simulink model "Model_Slides"  (R2021b)
settings: Solver=VariableStepAuto  StartTime=0.0  StopTime=inf  RelTol=1e-3
model workspace (MAT data in the model file):
  firstWarning = 1
  originalScenarioChecksum = '114339432DE22364D47BB28FC96DC10C'
undefined symbols (not defined in the file): Acceleration, ActorID, AngularVelocity, curvature, DefaultGear, DEND_B, DEND_S, DEND_T, direction, driving, gradbp, LF, LR, matlabshared, MAX_BRAKE, MAX_STEER, MAX_TORQUE, MCAR, MIN_BRAKE, MIN_STEER, MIN_TORQUE, NUMD_B, NUMD_S, NUMD_T, Pitch, Position, psi_o, R, Roll, RRdamp, scenario, SceneInfo, sigbuilder_block, STEER_RATIO, stopSign_ID, Tdead, thetaRefs, TL_ID, TrackWidth, Ts, ts, Vdead, Velocity, X_o, xRef2s, Y_o, Yaw, yRef2s
libraries: drivingscenarioandsensors x8, drivingvehiclecontroller x2, simulink x2, trackingutilitieslib x2, mpcadaslib x1, simulink_extras x1, drivinglib x1, autolibshared x1, vehdynlibviscommon x1, vehdynlibsteering x1
(part 1 of 2)
settings Model: Creator=akshran  LastModifiedBy=moham

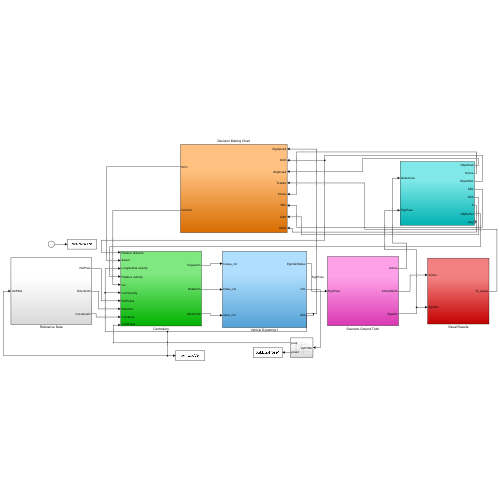
[thumbnail: Simulink's stored preview of the top-level diagram]
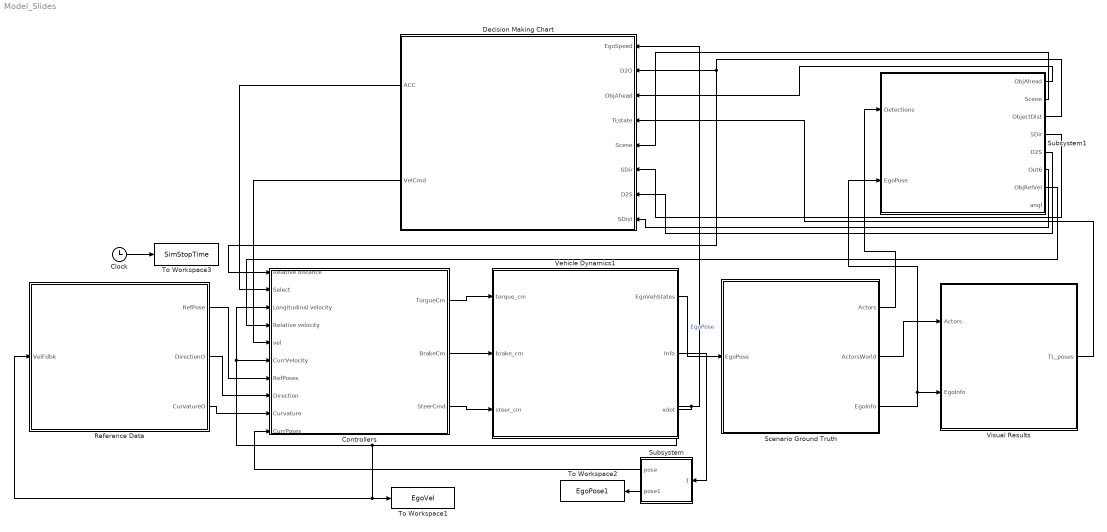
== system Model_Slides ==
  Clock : Clock
  Controllers : Subsystem
  Decision Making Chart : Subsystem
  Reference Data : Subsystem  VariantControl=Stanley
  Scenario Ground Truth : Subsystem
  Subsystem : Subsystem
  Subsystem1 : Subsystem
  To Workspace1 : ToWorkspace  VariableName=EgoVel  SampleTime=-1
      settings: Save2DSignal=2-D array (concatenate along first dimension)
  To Workspace2 : ToWorkspace  VariableName=EgoPose1  SampleTime=-1
      settings: Save2DSignal=2-D array (concatenate along first dimension)
  To Workspace3 : ToWorkspace  VariableName=SimStopTime  SampleTime=-1
      settings: Save2DSignal=2-D array (concatenate along first dimension)
  Vehicle Dynamics1 : Subsystem
  Visual Results : Subsystem
  wires:
  Vehicle Dynamics1/2(Info) -> Subsystem/1(VehFdbk)
  Clock/1 -> To Workspace3/1
  Vehicle Dynamics1/3(xdot) -> Reference Data/1(VelFdbk), To Workspace1/1, Controllers/6(CurrVelocity), Controllers/3(Longitudinal velocity), Decision Making Chart/1(EgoSpeed)
  Subsystem/2(pose1) -> To Workspace2/1
  Reference Data/1(RefPose) -> Controllers/7(RefPoses)
  Reference Data/2(DirectionO) -> Controllers/8(Direction)
  Reference Data/3(CurvatureO) -> Controllers/9(Curvature)
  Subsystem/1(pose) -> Controllers/10(CurrPoses)
  Controllers/1(TorgueCm) -> Vehicle Dynamics1/1(torque_cm)
  Controllers/2(BrakeCm) -> Vehicle Dynamics1/2(brake_cm)
  Controllers/3(SteerCmd) -> Vehicle Dynamics1/3(steer_cm)
  Visual Results/1(TL_poses) -> Decision Making Chart/4(TLstate)
  Decision Making Chart/1(ACC) -> Controllers/2(Select)
  Decision Making Chart/2(VelCmd) -> Controllers/5(vel)
  Subsystem1/3(ObjectDist) -> Controllers/1(Relative distance), Decision Making Chart/2(D2O)
  Subsystem1/1(ObjAhead) -> Decision Making Chart/3(ObjAhead)
  Subsystem1/2(Scene) -> Decision Making Chart/5(Scene)
  Subsystem1/4(SDir) -> Decision Making Chart/6(SDir)
  Subsystem1/5(D2S) -> Decision Making Chart/7(D2S)
  Subsystem1/6(Out6) -> Decision Making Chart/8(SDist)
  Subsystem1/7(ObjRelVel) -> Controllers/4(Relative velocity)
  Vehicle Dynamics1/1(EgoVehStates) -> Scenario Ground Truth/1(EgoPose)  "EgoPose"
  Scenario Ground Truth/1(Actors) -> Subsystem1/1(Detections)
  Scenario Ground Truth/2(ActorsWorld) -> Visual Results/1(Actors)
  Scenario Ground Truth/3(EgoInfo) -> Subsystem1/2(EgoPose), Visual Results/2(EgoInfo)

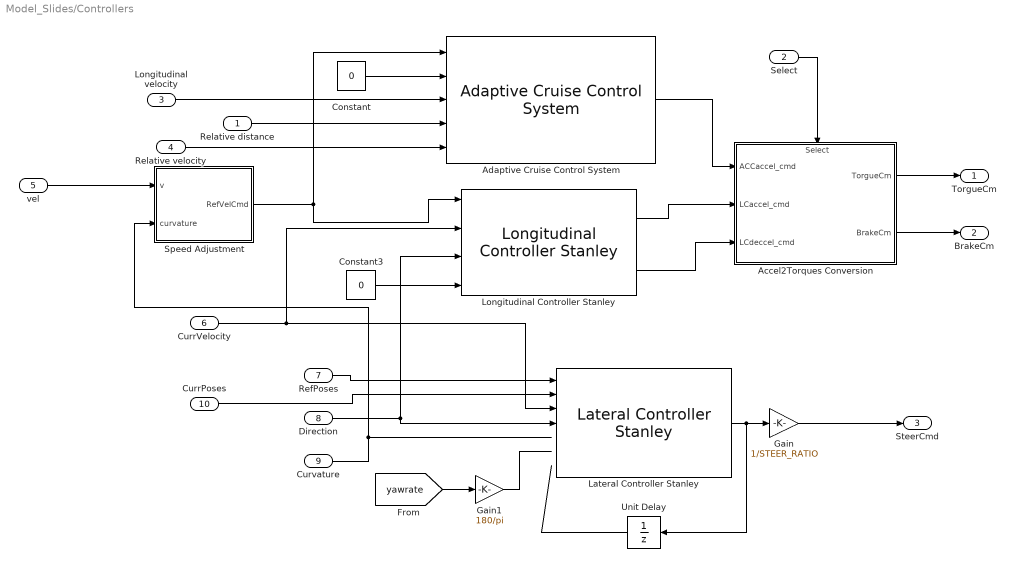
== system Model_Slides/Controllers ==
  Relative distance : Inport
  Select : Inport  Port=2
  Longitudinal velocity : Inport  Port=3
  Relative velocity : Inport  Port=4
  vel : Inport  Port=5
  CurrVelocity : Inport  Port=6
  RefPoses : Inport  Port=7
  Direction : Inport  Port=8
  Curvature : Inport  Port=9
  CurrPoses : Inport  Port=10
  Accel2Torques Conversion : Subsystem
      settings: PortSchema="{\"entries\":[{\"content\":{\"sides\":[{\"content\":{\"connectorIds\":[\"In1\",\"In2\",\"In3\"]},\"type\":\"ConnectorPlacement.EquallySpacedRectSide\",\"uuid\":\"a23b1a10-3bcb-40a0-900c-c9a3f160b173\"},{\"content\":{\"connectorIds\":[\"Out1\",\"Out2\"],\"side\":\"RIGHT\"},\"type\":\"ConnectorPlacement.EquallySpacedRectSide\",\"uuid\":\"88840b66-912f-4184-aeec-297642319416\"},{\"content\":{\"connectorIds\":[\"In4\"],\"side\":\"TOP\"},\"type\":\"ConnectorPlacement.EquallySpacedRectSide\",\"uuid\":\"37a03ca9-b065-473e-b290-3b07703c6005\"}]},\"type\":\"ConnectorPlacement.EquallySpacedConnector\",\"uuid\":\"5bfc7c71-8f7a-4cba-a168-7eeca22a2fcb\"}],\"packageUris\":[\"http://schema.mathworks.com/mf0/Connector/R2020b\"],\"version\":\"1.0\"}"
  Adaptive Cruise Control System : mpcadaslib/Adaptive Cruise Control System  EgoModel=tf(1,[0.5,1,0])  InitialEgoVelocity=0  DefaultSpacing=10  MaxVelocity=50  MinAcceleration=-6  amin_ext=off  MaxAcceleration=6  amax_ext=off  Ts=0.1  PredictionHorizon=30  ControllerBehavior=0.5  suboptimal=off  maxiter=10  datatypeopt=double  optmode=off  trackmode=off
  Constant : Constant  Value=0
  Constant3 : Constant  Value=0
  Gain : Gain  Gain=1/STEER_RATIO
  Gain1 : Gain  Gain=180/pi
  Lateral Controller Stanley : drivingvehiclecontroller/Lateral Controller Stanley  ModelType=Dynamic bicycle model  PositionGainF=2.5  PositionGainR=2.5  YawRateGain=0.2  DelayGain=0.2  VehicleMass=MCAR  Lf=LF  Lr=LR  TireStiffness=5e3  Wheelbase=3  MaxSteeringAngle=80
      settings: SourceProductBaseCode=DR
  Longitudinal Controller Stanley : drivingvehiclecontroller/Longitudinal Controller Stanley  Kp=10  Ki=0.1  SampleTime=0.05  MaxAcceleration=40  MaxDeceleration=40
      settings: SourceProductBaseCode=DR
  Speed Adjustment : MATLAB Function  TreatAsAtomicUnit=on
  Unit Delay : UnitDelay  SampleTime=-1  HasFrameUpgradeWarning=on
  TorgueCm : Outport
  BrakeCm : Outport  Port=2
  SteerCmd : Outport  Port=3
  wires:
  Gain1/1 -> ?
  Adaptive Cruise Control System/1 -> Accel2Torques Conversion/1(ACCaccel_cmd)
  Speed Adjustment/1(RefVelCmd) -> Adaptive Cruise Control System/1, Longitudinal Controller Stanley/1
  Curvature/1 -> Speed Adjustment/2(curvature)
  Unit Delay/1 -> ?
  Direction/1 -> Lateral Controller Stanley/4, Longitudinal Controller Stanley/3
  Lateral Controller Stanley/1 -> Unit Delay/1, Gain/1
  Longitudinal Controller Stanley/2 -> Accel2Torques Conversion/3(LCdeccel_cmd)
  Relative distance/1 -> Adaptive Cruise Control System/4
  Constant/1 -> Adaptive Cruise Control System/2
  [yawrate] -> Gain1/1
  Constant3/1 -> Longitudinal Controller Stanley/4
  Longitudinal Controller Stanley/1 -> Accel2Torques Conversion/2(LCaccel_cmd)
  CurrPoses/1 -> Lateral Controller Stanley/2
  RefPoses/1 -> Lateral Controller Stanley/1
  Gain/1 -> SteerCmd/1
  Longitudinal velocity/1 -> Adaptive Cruise Control System/3
  Select/1 -> Accel2Torques Conversion/4(Select)
  Relative velocity/1 -> Adaptive Cruise Control System/5
  Accel2Torques Conversion/2(BrakeCm) -> BrakeCm/1
  Accel2Torques Conversion/1(TorgueCm) -> TorgueCm/1
  vel/1 -> Speed Adjustment/1(v)
  CurrVelocity/1 -> Lateral Controller Stanley/3, Longitudinal Controller Stanley/2

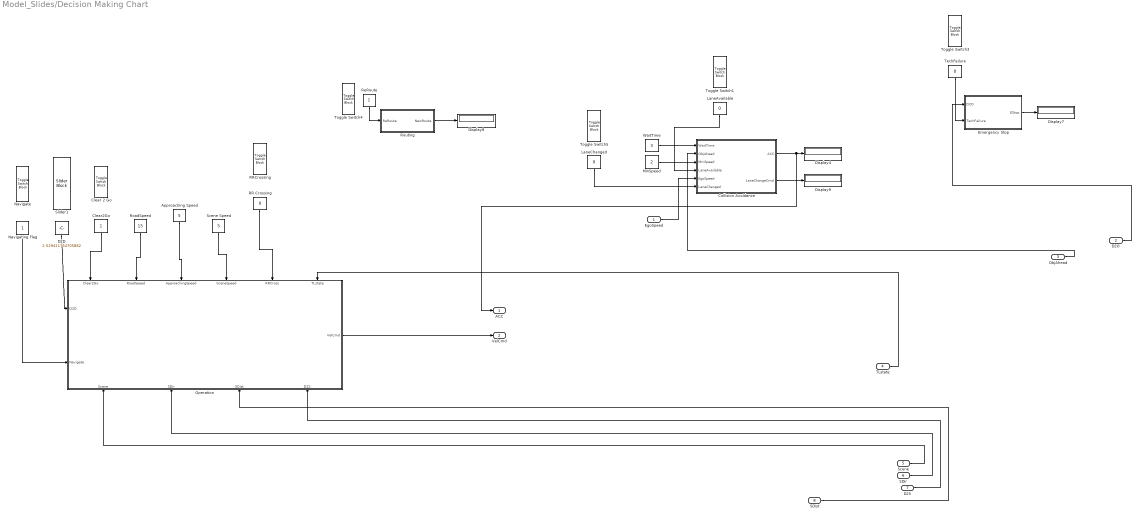
== system Model_Slides/Decision Making Chart ==
  EgoSpeed : Inport
  D2O : Inport  Port=2
  ObjAhead : Inport  Port=3
  TLstate : Inport  Port=4
  Scene : Inport  Port=5
  SDir : Inport  Port=6
  D2S : Inport  Port=7
  SDist : Inport  Port=8
  Approaching Speed : Constant  Value=5
  Clear 2 Go : ToggleSwitchBlock
      settings: Values={{'Off', 'On'}, [0 1]}
  Clear2Go : Constant
  Collision Avoidance : Stateflow chart  TreatAsAtomicUnit=on
  D2D : Constant  Value=2.529411764705882
  Display{4,7..9} (4 alike) : Display
  Emergency Stop : Stateflow chart  TreatAsAtomicUnit=on
  LaneAvailable : Constant  Value=0
  LaneChanged : Constant  Value=0
  MinSpeed : Constant  Value=2
  Navigate : ToggleSwitchBlock
      settings: Values={{'Off', 'On'}, [0 1]}
  Navigating Flag : Constant
  Operation : Stateflow chart  TreatAsAtomicUnit=on
      settings: PortSchema="{\"entries\":[{\"content\":{\"sides\":[{\"content\":{\"connectorIds\":[\"In10\",\"In9\"]},\"type\":\"ConnectorPlacement.EquallySpacedRectSide\",\"uuid\":\"81aca70f-0947-49fb-b60a-be241e44193b\"},{\"content\":{\"connectorIds\":[\"Out1\"],\"side\":\"RIGHT\"},\"type\":\"ConnectorPlacement.EquallySpacedRectSide\",\"uuid\":\"e7b9645e-3711-4964-ac9b-0199dd335e99\"},{\"content\":{\"connectorIds\":[\"In11\",\"In12\",\"In3\",\"In4\",\"In6\",\"In1\"],\"side\":\"TOP\"},\"type\":\"ConnectorPlacement.EquallySpacedRectSide\",\"uuid\":\"6876f024-944b-4540-9404-d68f37763657\"},{\"content\":{\"connectorIds\":[\"In8\",\"In2\",\"In5\",\"In7\"],\"side\":\"BOTTOM\"},\"type\":\"ConnectorPlacement.EquallySpacedRectSide\",\"uuid\":\"44acab73-cdde-4edf-95df-27422644ccab\"}]},\"type\":\"ConnectorPlacement.EquallySpacedConnector\",\"uuid\":\"d2c31c01-e447-43db-8d2b-8b98a0ca291a\"}],\"packageUris\":[\"http://schema.mathworks.com/mf0/Connector/R2020b\"],\"version\":\"1.0\"}"
  RR Crossing : Constant  Value=0
  RRCrossing : ToggleSwitchBlock
      settings: Values={{'Off', 'On'}, [0 1]}
  ReRoute : Constant
  RoadSpeed : Constant  Value=15
  Routing : Stateflow chart  TreatAsAtomicUnit=on
  Scene Speed : Constant  Value=5
  Slider1 : SliderBlock  ScaleMax=5
  TechFailure : Constant  Value=0
  Toggle Switch{1,3..5} (4 alike) : ToggleSwitchBlock
      settings: Values={{'Off', 'On'}, [0 1]}
  WaitTime : Constant  Value=3
  ACC : Outport
  VelCmd : Outport  Port=2
  wires:
  Collision Avoidance/1(ACC) -> ACC/1, Display4/1
  ObjAhead/1 -> Collision Avoidance/2(ObjAhead)
  D2S/1 -> Operation/7(D2S)
  D2D/1 -> Operation/10(D2D)
  Clear2Go/1 -> Operation/11(Clear2Go)
  RoadSpeed/1 -> Operation/12(RoadSpeed)
  SDir/1 -> Operation/2(SDir)
  RR Crossing/1 -> Operation/6(RRCross)
  Approaching Speed/1 -> Operation/3(ApproachingSpeed)
  TechFailure/1 -> Emergency Stop/2(TechFailure)
  WaitTime/1 -> Collision Avoidance/1(WaitTime)
  Scene/1 -> Operation/8(Scene)
  Navigating Flag/1 -> Operation/9(Navigate)
  LaneAvailable/1 -> Collision Avoidance/4(LaneAvailable)
  ReRoute/1 -> Routing/1(ReRoute)
  LaneChanged/1 -> Collision Avoidance/6(LaneChanged)
  Operation/1(VelCmd) -> VelCmd/1
  Scene Speed/1 -> Operation/4(SceneSpeed)
  TLstate/1 -> Operation/1(TLstate)
  Collision Avoidance/2(LaneChangeCmd) -> Display9/1
  Emergency Stop/1(EStop) -> Display7/1
  MinSpeed/1 -> Collision Avoidance/3(MinSpeed)
  Routing/1(NewRoute) -> Display8/1
  SDist/1 -> Operation/5(SDist)
  EgoSpeed/1 -> Collision Avoidance/5(EgoSpeed)
  D2O/1 -> Emergency Stop/1(D2O)

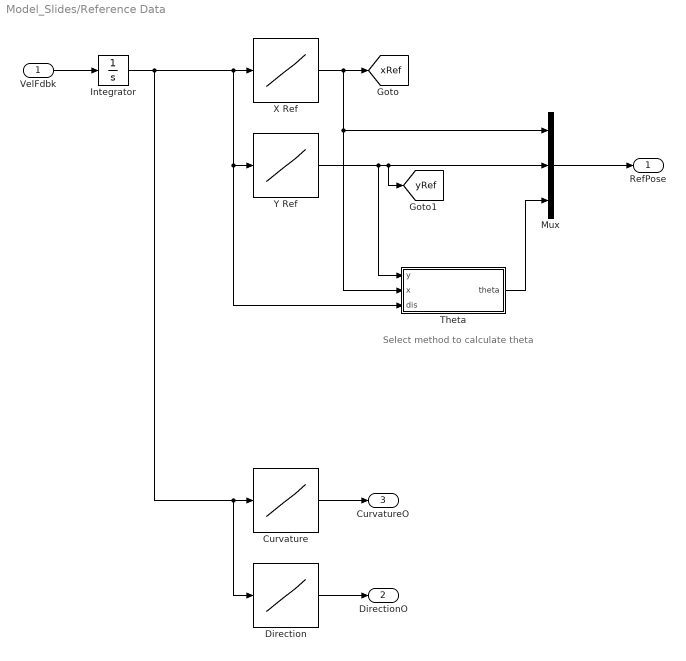
== system Model_Slides/Reference Data ==
  note: Select method to calculate theta
  VelFdbk : Inport
  Curvature : Lookup_n-D  NumberOfTableDimensions=1  BreakpointsForDimension1=gradbp  Table=curvature  InternalRulePriority=Speed  RndMeth=Simplest  InputSameDT=on
  Direction : Lookup_n-D  NumberOfTableDimensions=1  BreakpointsForDimension1=gradbp  Table=direction  InternalRulePriority=Speed  RndMeth=Simplest  InputSameDT=on
  Integrator : Integrator
  Mux : Mux  Inputs=3
  Theta : Subsystem  Variant=on  VariantControlMode=label  LabelModeActiveChoice=thetaSimulinkBlock
  X Ref : Lookup_n-D  NumberOfTableDimensions=1  BreakpointsForDimension1=gradbp  Table=xRef2s  InternalRulePriority=Speed  RndMeth=Simplest  InputSameDT=on
  Y Ref : Lookup_n-D  NumberOfTableDimensions=1  BreakpointsForDimension1=gradbp  Table=yRef2s  InternalRulePriority=Speed  RndMeth=Simplest  InputSameDT=on
  RefPose : Outport
  DirectionO : Outport  Port=2
  CurvatureO : Outport  Port=3
  tag scope: xRef=global, yRef=global
  wires:
  Direction/1 -> DirectionO/1
  Curvature/1 -> CurvatureO/1
  Y Ref/1 -> Theta/1(y), Mux/2, [yRef]
  Mux/1 -> RefPose/1
  X Ref/1 -> Theta/2(x), Mux/1, [xRef]
  Integrator/1 -> Curvature/1, Direction/1, Theta/3(dis), Y Ref/1, X Ref/1
  VelFdbk/1 -> Integrator/1
  Theta/1(theta) -> Mux/3

== system Model_Slides/Scenario Ground Truth ==
  EgoPose : Inport
  Scenario Reader : drivingscenarioandsensors/Scenario Reader  ScenarioSource=From file  ScenarioFileName=C:\Users\moham\MATLAB Drive\AutoDrive Challenge II\ad2_y1_simulationpkg_(2)\ad2_y1_simulationpkg\scenarios\scenario_SS_TL_junction.mat  ScenarioVariableName=scenario  OutputCoordinateSystem=Vehicle coordinates  EgoVehicleSource=Input port  EgoVehicleActorID=1  OrientVehiclesOnRoad=on  OutputEgoVehiclePose=on  OutputEgoVehicleState=off  SampleTime=Ts  LaneBoundaryOutput=None  LaneBoundaryDistance=0:0.5:9.5  LaneBoundaryLocation=Center of lane markings  BusNameSource=Auto  BusName=BusActors  BusNumActorsSource=Scenario  BusNumActors=100  BusName2Source=Auto  BusName2=BusLaneBoundaries  BusNumLaneBoundariesSource=Scenario  BusNumLaneBoundaries=10  BusName3Source=Auto  BusName3=BusEgoActor  BusName4Source=Auto  BusName4=BusEgoState  ShowCoordinateLabels=on  SimulateUsing=Interpreted execution
  To Workspace : ToWorkspace  VariableName=EgoPose  SaveFormat=Timeseries  SampleTime=-1
  Vehicle To World : drivingscenarioandsensors/Vehicle To World  BusNameSource=Auto  BusName=BusVehicleToWorldActors  SimulateUsing=Interpreted execution
      settings: SourceProductBaseCode=DR
  Actors : Outport
  ActorsWorld : Outport  Port=2
  EgoInfo : Outport  Port=3
  wires:
  Scenario Reader/1 -> Actors/1, Vehicle To World/1  "Actors"
  EgoPose/1 -> EgoInfo/1, Vehicle To World/2, To Workspace/1, Scenario Reader/1
  Vehicle To World/1 -> ActorsWorld/1  "ActorsWorld"

== system Model_Slides/Subsystem ==
  VehFdbk : Inport
  Bus Selector : BusSelector  OutputSignals=InertFrm.Cg.Disp.X,InertFrm.Cg.Disp.Y,InertFrm.Cg.Ang.psi
  Bus Selector1 : BusSelector  OutputSignals=InertFrm.Cg.Disp.X,InertFrm.Cg.Disp.Y,InertFrm.Cg.Disp.Z
  Gain1 : Gain  Gain=180/pi
  Mux : Mux  Inputs=3
  Mux1 : Mux  Inputs=3
  Transpose : Math  Operator=transpose  SignedPower=on  SaturateOnIntegerOverflow=on
  Transpose1 : Math  Operator=transpose  SignedPower=on  SaturateOnIntegerOverflow=on
  pose : Outport
  pose1 : Outport  Port=2
  wires:
  Mux/1 -> Transpose/1
  VehFdbk/1 -> Bus Selector1/1, Bus Selector/1
  Bus Selector/1 -> Mux/1  "<X>"
  Gain1/1 -> Mux/3
  Bus Selector/2 -> Mux/2  "<Y>"
  Transpose/1 -> pose/1
  Bus Selector/3 -> Gain1/1  "<psi>"
  Bus Selector1/1 -> Mux1/1  "<X>"
  Bus Selector1/2 -> Mux1/2  "<Y>"
  Bus Selector1/3 -> Mux1/3  "<Z>"
  Mux1/1 -> Transpose1/1
  Transpose1/1 -> pose1/1

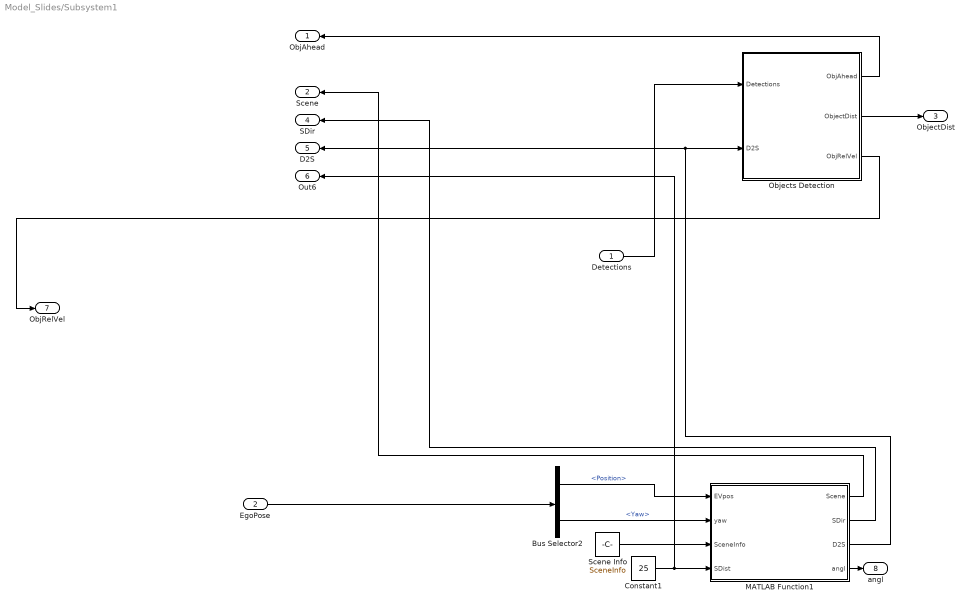
== system Model_Slides/Subsystem1 ==
  Detections : Inport
  EgoPose : Inport  Port=2
  Bus Selector2 : BusSelector  OutputSignals=Position,Yaw
  Constant1 : Constant  Value=25
  MATLAB Function1 : MATLAB Function  TreatAsAtomicUnit=on
  Objects Detection : Subsystem
  Scene Info : Constant  Value=SceneInfo  VectorParams1D=off
  ObjAhead : Outport
  Scene : Outport  Port=2
  ObjectDist : Outport  Port=3
  SDir : Outport  Port=4
  D2S : Outport  Port=5
  Out6 : Outport  Port=6
  ObjRelVel : Outport  Port=7
  angl : Outport  Port=8
  wires:
  Objects Detection/2(ObjectDist) -> ObjectDist/1
  MATLAB Function1/3(D2S) -> D2S/1, Objects Detection/2(D2S)
  MATLAB Function1/4(angl) -> angl/1
  Constant1/1 -> Out6/1, MATLAB Function1/4(SDist)
  Scene Info/1 -> MATLAB Function1/3(SceneInfo)
  EgoPose/1 -> Bus Selector2/1
  Bus Selector2/1 -> MATLAB Function1/1(EVpos)  "<Position>"
  Bus Selector2/2 -> MATLAB Function1/2(yaw)  "<Yaw>"
  Detections/1 -> Objects Detection/1(Detections)
  MATLAB Function1/1(Scene) -> Scene/1
  MATLAB Function1/2(SDir) -> SDir/1
  Objects Detection/3(ObjRelVel) -> ObjRelVel/1
  Objects Detection/1(ObjAhead) -> ObjAhead/1

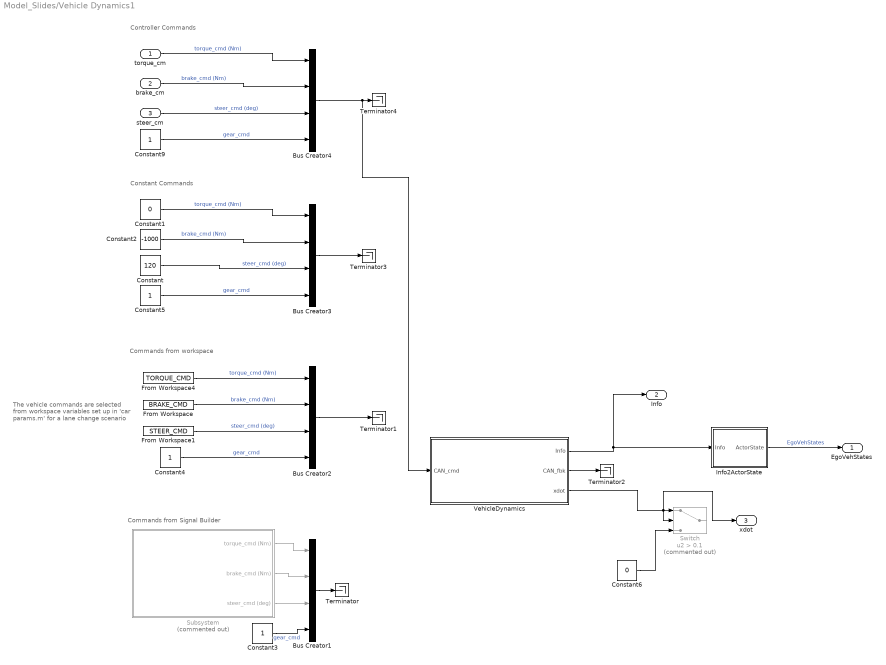
== system Model_Slides/Vehicle Dynamics1 ==
  note: Constant Commands
  note: Commands from workspace
  note: Commands from Signal Builder
  note: The vehicle commands are selected from workspace variables set up in 'car params.m' for a lane change scenario
  note: Controller Commands
  torque_cm : Inport
  brake_cm : Inport  Port=2
  steer_cm : Inport  Port=3
  Bus Creator{1..4} (4 alike) : BusCreator  Inputs=4
  Constant : Constant  Value=120
  Constant1 : Constant  Value=0
  Constant2 : Constant  Value=-1000
  Constant{3..5,9} (4 alike) : Constant
  Constant6 : Constant  Value=0
  From Workspace : FromWorkspace  VariableName=BRAKE_CMD  SampleTime=ts
  From Workspace1 : FromWorkspace  VariableName=STEER_CMD  SampleTime=ts
  From Workspace4 : FromWorkspace  VariableName=TORQUE_CMD  SampleTime=ts
  Info2ActorState : Subsystem
  Subsystem : Subsystem  Commented=on
  Switch : Switch  Commented=on  Criteria=u2 > Threshold  Threshold=0.1
  Terminator{,1..4} (5 alike) : Terminator
  VehicleDynamics : Subsystem  mask{InitPosition=scenario.Actors(1).Position-0.5*scenario.Actors(1).Wheelbase*[cosd(scenario.Actors(1).Yaw) sind(scenario.Actors(1).Yaw) 0], InitSpeed=norm(scenario.Actors(1).Velocity)*0, InitYaw=(scenario.Actors(1).Yaw/scenario.Actors(1).Yaw)*psi_o}
      mask prompts: InitPosition "Initial Position (m)"; InitSpeed "Initial Speed (m/s)"; InitYaw "Init Yaw (rad)"
  EgoVehStates : Outport
  Info : Outport  Port=2
  xdot : Outport  Port=3
  wires:
  Bus Creator2/1 -> Terminator1/1
  VehicleDynamics/2(CAN_fbk) -> Terminator2/1
  VehicleDynamics/1(Info) -> Info/1, Info2ActorState/1(Info)
  Constant/1 -> Bus Creator3/3  "steer_cmd (deg)"
  Info2ActorState/1(ActorState) -> EgoVehStates/1  "EgoVehStates"
  Constant1/1 -> Bus Creator3/1  "torque_cmd (Nm)"
  Constant2/1 -> Bus Creator3/2  "brake_cmd (Nm)"
  VehicleDynamics/3(xdot) -> Switch/2, Switch/1, xdot/1
  Subsystem/1(torque_cmd (Nm)) -> Bus Creator1/1
  Subsystem/2(brake_cmd (Nm)) -> Bus Creator1/2
  Subsystem/3(steer_cmd (deg)) -> Bus Creator1/3
  Constant3/1 -> Bus Creator1/4  "gear_cmd"
  Constant4/1 -> Bus Creator2/4  "gear_cmd"
  From Workspace/1 -> Bus Creator2/2  "brake_cmd (Nm)"
  From Workspace1/1 -> Bus Creator2/3  "steer_cmd (deg)"
  From Workspace4/1 -> Bus Creator2/1  "torque_cmd (Nm)"
  Constant5/1 -> Bus Creator3/4  "gear_cmd"
  Bus Creator1/1 -> Terminator/1
  brake_cm/1 -> Bus Creator4/2  "brake_cmd (Nm)"
  Constant9/1 -> Bus Creator4/4  "gear_cmd"
  torque_cm/1 -> Bus Creator4/1  "torque_cmd (Nm)"
  steer_cm/1 -> Bus Creator4/3  "steer_cmd (deg)"
  Bus Creator3/1 -> Terminator3/1
  Bus Creator4/1 -> VehicleDynamics/1(CAN_cmd), Terminator4/1
  Constant6/1 -> Switch/3

== system Model_Slides/Visual Results ==
  note: Traffic Lights and Stop Signs
  Actors : Inport
  EgoInfo : Inport  Port=2
  Bus Selector : BusSelector  OutputSignals=Actors
  Lights and Signs ID : Subsystem
  "Positions and States " : Subsystem
  Visualization : Subsystem
  TL_poses : Outport
  wires:
  "Positions and States "/1(TL_poses) -> TL_poses/1, Visualization/1(TL1_poses)
  Actors/1 -> Visualization/2(Actors), Bus Selector/1
  Lights and Signs ID/2(Stop_Sign) -> "Positions and States "/3(ss_State)
  Lights and Signs ID/1(TL) -> "Positions and States "/2(TL_id)
  Bus Selector/1 -> "Positions and States "/1(<Actors>)  "<Actors>"
  "Positions and States "/2(ss_poses) -> Visualization/4(ss1_poses)
  EgoInfo/1 -> Visualization/3(EgoInfo)

== system Model_Slides/Controllers/Accel2Torques Conversion ==
  ACCaccel_cmd : Inport
  LCaccel_cmd : Inport  Port=2
  LCdeccel_cmd : Inport  Port=3
  Select : Inport  Port=4
  Merge1 : Merge
  Merge2 : Merge
  Subsystem1 : Subsystem
  Subsystem2 : Subsystem
  Switch Case1 : SwitchCase  CaseConditions={1, 0}  ShowDefaultCase=off
  TorgueCm : Outport
  BrakeCm : Outport  Port=2
  wires:
  LCdeccel_cmd/1 -> Subsystem1/2(decc_cmd)
  Subsystem1/2(brake_cm) -> Merge2/2
  Subsystem1/1(torque_cm) -> Merge1/2
  Subsystem2/2(brake_cm) -> Merge2/1
  Switch Case1/1 -> Subsystem2/Action
  Switch Case1/2 -> Subsystem1/Action
  Subsystem2/1(torque_cm) -> Merge1/1
  LCaccel_cmd/1 -> Subsystem1/1(acc_cmd)
  Merge2/1 -> BrakeCm/1
  ACCaccel_cmd/1 -> Subsystem2/1(acc_cmd)
  Merge1/1 -> TorgueCm/1
  Select/1 -> Switch Case1/1

== system Model_Slides/Reference Data/Theta ==
  note: 1) Add Subsystem or Model blocks as valid variant choices.
      | 2) You cannot connect blocks at this level. At simulation, connectivity is automatically
      | determined, based on the active variant and port name matching.
  y : Inport
  x : Inport  Port=2
  dis : Inport  Port=3
  thetaBlocks : Subsystem  VariantControl=thetaSimulinkBlock
  thetaLt : Subsystem  VariantControl=thetaLookUpTable
  theta : Outport

== system Model_Slides/Subsystem1/Objects Detection ==
  Detections : Inport
  D2S : Inport  Port=2
  MATLAB Function : MATLAB Function  TreatAsAtomicUnit=on
  Terminator1 : Terminator
  Terminator2 : Terminator
  Tracking : Subsystem
  ObjAhead : Outport
  ObjectDist : Outport  Port=2
  ObjRelVel : Outport  Port=3
  wires:
  MATLAB Function/4(ObjectDist) -> ObjectDist/1
  MATLAB Function/2(TracksNum) -> Terminator2/1
  Tracking/1(Confirmed_Tracks) -> MATLAB Function/2(Tracking)
  Detections/1 -> Tracking/1(Detections)
  MATLAB Function/1(ObjectID) -> Terminator1/1
  MATLAB Function/5(ObjAhead) -> ObjAhead/1
  D2S/1 -> MATLAB Function/1(D2S)
  MATLAB Function/3(ObjRelVel) -> ObjRelVel/1

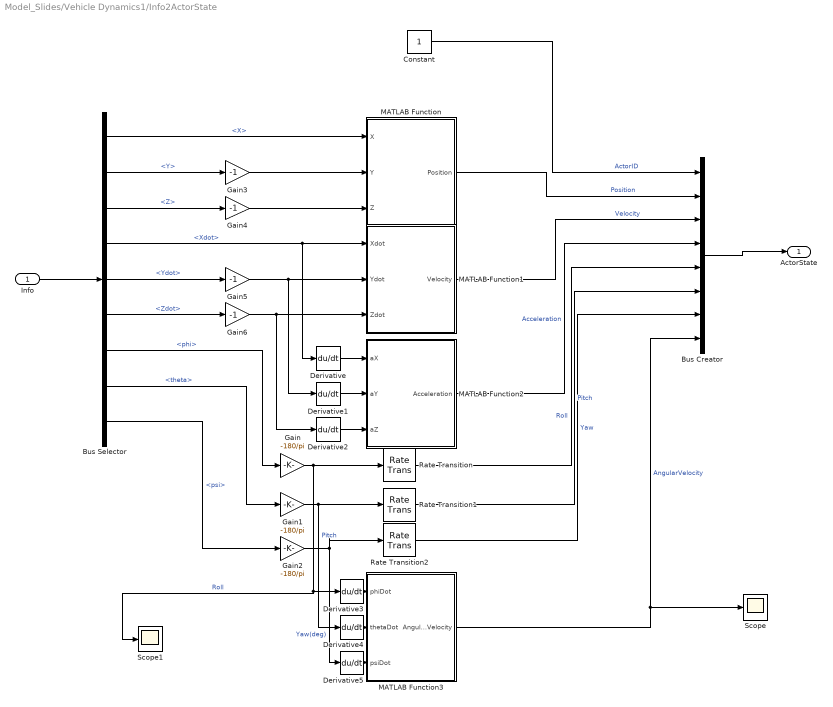
== system Model_Slides/Vehicle Dynamics1/Info2ActorState ==
  Info : Inport
  Bus Creator : BusCreator  Inputs=ActorID,Position,Velocity,Acceleration,Roll,Pitch,Yaw,AngularVelocity  OutDataTypeStr=Bus: BusActorState  NonVirtualBus=on
  Bus Selector : BusSelector  OutputSignals=InertFrm.Cg.Disp.X,InertFrm.Cg.Disp.Y,InertFrm.Cg.Disp.Z,InertFrm.Cg.Vel.Xdot,InertFrm.Cg.Vel.Ydot,InertFrm.Cg.Vel.Zdot,InertFrm.Cg.Ang.phi,InertFrm.Cg.Ang.theta,InertFrm.Cg.Ang.psi
  Constant : Constant  SampleTime=0.05
  Derivative{,1..5} (6 alike) : Derivative
  Gain : Gain  Gain=-180/pi
  Gain1 : Gain  Gain=-180/pi
  Gain2 : Gain  Gain=-180/pi
  Gain{3..6} (4 alike) : Gain  Gain=-1
  MATLAB Function : MATLAB Function  TreatAsAtomicUnit=on  SystemSampleTime=0.05
  MATLAB Function1 : MATLAB Function  TreatAsAtomicUnit=on  SystemSampleTime=0.05
  MATLAB Function2 : MATLAB Function  TreatAsAtomicUnit=on  SystemSampleTime=0.05
  MATLAB Function3 : MATLAB Function  TreatAsAtomicUnit=on  SystemSampleTime=0.05
  Rate Transition : RateTransition  OutPortSampleTime=0.05
  Rate Transition1 : RateTransition  OutPortSampleTime=0.05
  Rate Transition2 : RateTransition  OutPortSampleTime=0.05
  Scope : Scope
  Scope1 : Scope
  ActorState : Outport
  wires:
  Gain/1 -> Scope1/1, Derivative3/1, Rate Transition/1  "Roll"
  Derivative4/1 -> MATLAB Function3/2(thetaDot)
  Bus Selector/2 -> Gain3/1  "<Y>"
  Bus Selector/4 -> Derivative/1, MATLAB Function1/1(Xdot)  "<Xdot>"
  MATLAB Function1/1(Velocity) -> Bus Creator/3  "Velocity"
  MATLAB Function/1(Position) -> Bus Creator/2  "Position"
  Derivative1/1 -> MATLAB Function2/2(aY)
  Bus Selector/5 -> Gain5/1  "<Ydot>"
  Bus Selector/1 -> MATLAB Function/1(X)  "<X>"
  Bus Selector/9 -> Gain2/1  "<psi>"
  Gain2/1 -> Rate Transition2/1, Derivative5/1  "Yaw(deg)"
  Derivative5/1 -> MATLAB Function3/3(psiDot)
  Bus Selector/7 -> Gain/1  "<phi>"
  MATLAB Function2/1(Acceleration) -> Bus Creator/4  "Acceleration"
  Derivative3/1 -> MATLAB Function3/1(phiDot)
  Gain1/1 -> Derivative4/1, Rate Transition1/1  "Pitch"
  Bus Selector/6 -> Gain6/1  "<Zdot>"
  Bus Selector/8 -> Gain1/1  "<theta>"
  MATLAB Function3/1(AngularVelocity) -> Bus Creator/8, Scope/1  "AngularVelocity"
  Bus Selector/3 -> Gain4/1  "<Z>"
  Derivative2/1 -> MATLAB Function2/3(aZ)
  Derivative/1 -> MATLAB Function2/1(aX)
  Info/1 -> Bus Selector/1
  Constant/1 -> Bus Creator/1  "ActorID"
  Bus Creator/1 -> ActorState/1
  Rate Transition/1 -> Bus Creator/5  "Roll"
  Rate Transition1/1 -> Bus Creator/6  "Pitch"
  Rate Transition2/1 -> Bus Creator/7  "Yaw"
  Gain3/1 -> MATLAB Function/2(Y)
  Gain4/1 -> MATLAB Function/3(Z)
  Gain5/1 -> Derivative1/1, MATLAB Function1/2(Ydot)
  Gain6/1 -> Derivative2/1, MATLAB Function1/3(Zdot)

== system Model_Slides/Vehicle Dynamics1/Subsystem ==
  Gain : Gain  Gain=MAX_TORQUE*0.1
  Gain1 : Gain  Gain=MIN_BRAKE*0.06
  Gain2 : Gain  Gain=MAX_STEER/4.5
  Signal Builder : Subsystem  Tag=STV Subsys  LoadFcn=sigbuilder_block('load');  StartFcn=sigbuilder_block('start');  StopFcn=sigbuilder_block('stop');  ClipboardFcn=sigbuilder_block('clipboard');  mask(Sigbuilder block){tuvar=[0:10]}
      mask help: Simulink:masks:SigbuilderBlock_MD
      mask init:
      | if ~strcmp(get_param(bdroot(gcbh),'SimulationStatus'),'stopped') tuvar = sigbuilder_block('maskInit'); end
      settings: CopyFcn=sigbuilder_block('copy');  DeleteFcn=sigbuilder_block('delete');  ModelCloseFcn=sigbuilder_block('modelClose');  PreSaveFcn=sigbuilder_block('preSave');  PauseFcn=sigbuilder_block('pause');  ContinueFcn=sigbuilder_block('continue');  NameChangeFcn=sigbuilder_block('namechange');  OpenFcn=sigbuilder_block('open',[0 30 960 455.5 ]);  CloseFcn=sigbuilder_block('close');
      mask Display: plot(0, 0, 100, 100,[2, 2, 32, 32, 2], [68, 8, 8, 68, 68],[32, 2], [38, 38], [32, 19, 2],[53, 60, 44], [32, 17, 17, 2],[16, 16, 31, 31]);txt = getActiveGroup(gcbh);text(2, 100, txt,'verticalAlignment', 'top');
  torque_cmd (Nm) : Outport
  brake_cmd (Nm) : Outport  Port=2
  steer_cmd (deg) : Outport  Port=3
  wires:
  Gain2/1 -> steer_cmd (deg)/1  "steer_cmd (deg)"
  Signal Builder/1(Normalized Torque) -> Gain/1
  Signal Builder/2(Normalized Brake) -> Gain1/1
  Signal Builder/3(Normalized Steer) -> Gain2/1  "steer_cmd (deg)"
  Gain1/1 -> brake_cmd (Nm)/1  "brake_cmd (Nm)"
  Gain/1 -> torque_cmd (Nm)/1  "torque_cmd (Nm)"

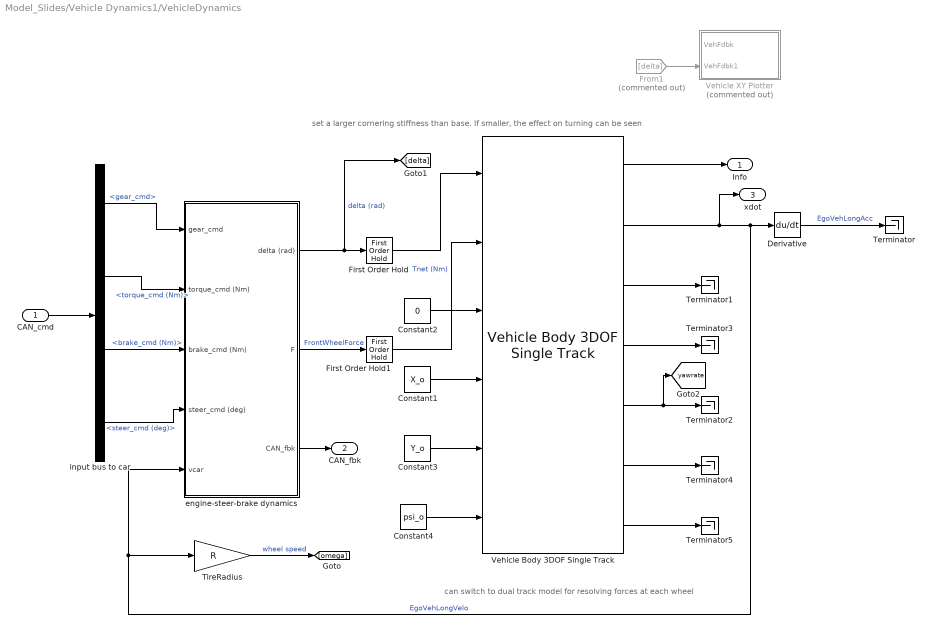
== system Model_Slides/Vehicle Dynamics1/VehicleDynamics ==
  note: set a larger cornering stiffness than base. If smaller, the effect on turning can be seen
  note: can switch to dual track model for resolving forces at each wheel
  CAN_cmd : Inport
  Constant1 : Constant  Value=X_o
  Constant2 : Constant  Value=0
  Constant3 : Constant  Value=Y_o
  Constant4 : Constant  Value=psi_o
  Derivative : Derivative
  First Order Hold : FirstOrderHold  ErrorTolerance=inf
  First Order Hold1 : FirstOrderHold  ErrorTolerance=inf
  From1 : From  Commented=on  GotoTag=delta
  Terminator{,1..5} (6 alike) : Terminator
  TireRadius : Gain  Gain=R
  Vehicle Body 3DOF Single Track : autolibshared/Vehicle Body 3DOF Single Track  trackMode=Single (bicycle)  inputMode=External longitudinal forces  frontSteerMode=on  rearSteerMode=off  windMode=off  muMode=off  extFMode=off  extMMode=off  htchFMode=off  htchMMode=off  extXo=on  extpsio=on  extxdoto=off  extro=off  extYo=on  extTamb=off  extydoto=off  aMode=2  NF=2  NR=2  m=MCAR  a=LF  b=LR  h=0.35  dh=1  hh=0.2  X_o=InitPosition(1)  xdot_o=InitSpeed  CalphaMode=off  sigmaMode=on  d=0  hl=0  w=[1.4,1.4]  Cy_f=12e3*100  Cy_r=11e3*100  sigma_f=.1  sigma_r=.1  alpha_f_brk=[-.1 .1]  Cy_f_data=[-9e3 9e3]  alpha_r_brk=[-.1 .1]  Cy_r_data=[-9e3 9e3]  Y_o=-InitPosition(2)  ydot_o=0  Izz=2050  psi_o=-InitYaw/180*pi  r_o=0  Af=2  Cd=.3  Cl=.1  Cpm=.1  beta_w=[0:0.01:0.3]  Cs=[0:0.03:0.9]  Cym=[0:0.01:0.3]  Pabs=101325  Tair=273  g=9.81  mu=1  xdot_tol=.01  Fznom=5000  Fxtire_sat=7e4  Fytire_sat=7e4  longOff=0  latOff=0  vertOff=0  wrapAng=off
      settings: SourceProductBaseCode=PW,DR,MT,UV,VE
  Vehicle XY Plotter : Subsystem  Commented=on  mask(Vehicle XY Plotter){a=LF, b=LR, w=TrackWidth, bufferSize=1024, pltDT=.1}
      mask prompts: a "Distance to front axle from CG, a [m]:"; b "Distance to rear axle from CG, b [m]:"; w "Track width, w [m]:"; bufferSize "Path buffer sampe size, bufferSize []:"; pltDT "Plot update rate, pltDT [s]:"
      mask help: This block will display a MATLAB figure which indicates the vehicle path, current position and heading velocity.
      mask TypeOptions a: Vehicle XY Plotter/a
      mask TypeOptions b: Vehicle XY Plotter/b
      mask TypeOptions w: Vehicle XY Plotter/w
      mask TypeOptions bufferSize: Vehicle XY Plotter/bufferSize
  engine-steer-brake dynamics : Subsystem
  input bus to car : BusSelector  OutputSignals=gear_cmd,torque_cmd (Nm),brake_cmd (Nm),steer_cmd (deg)
  Info : Outport
  CAN_fbk : Outport  Port=2  VectorParamsAs1DForOutWhenUnconnected=off
  xdot : Outport  Port=3
  tag scope: yawrate=global
  wires:
  TireRadius/1 -> [omega]  "wheel speed"
  Vehicle Body 3DOF Single Track/1 -> Info/1
  From1/1 -> Vehicle XY Plotter/2(VehFdbk1)
  input bus to car/1 -> engine-steer-brake dynamics/1(gear_cmd)  "<gear_cmd>"
  input bus to car/3 -> engine-steer-brake dynamics/3(brake_cmd (Nm))  "<brake_cmd (Nm)>"
  engine-steer-brake dynamics/1(delta (rad)) -> [delta], First Order Hold/1  "delta (rad)"
  input bus to car/2 -> engine-steer-brake dynamics/2(torque_cmd (Nm))  "<torque_cmd (Nm)>"
  input bus to car/4 -> engine-steer-brake dynamics/4(steer_cmd (deg))  "<steer_cmd (deg)>"
  engine-steer-brake dynamics/3(CAN_fbk) -> CAN_fbk/1
  CAN_cmd/1 -> input bus to car/1
  Constant2/1 -> Vehicle Body 3DOF Single Track/3
  engine-steer-brake dynamics/2(F) -> First Order Hold1/1  "FrontWheelForce"
  First Order Hold/1 -> Vehicle Body 3DOF Single Track/1
  Vehicle Body 3DOF Single Track/2 -> xdot/1, engine-steer-brake dynamics/5(vcar), TireRadius/1, Derivative/1  "EgoVehLongVelo"
  Vehicle Body 3DOF Single Track/3 -> Terminator1/1
  Vehicle Body 3DOF Single Track/4 -> Terminator3/1
  Vehicle Body 3DOF Single Track/5 -> [yawrate], Terminator2/1
  Vehicle Body 3DOF Single Track/6 -> Terminator4/1
  Vehicle Body 3DOF Single Track/7 -> Terminator5/1
  Derivative/1 -> Terminator/1  "EgoVehLongAcc"
  First Order Hold1/1 -> Vehicle Body 3DOF Single Track/2  "Tnet (Nm)"
  Constant1/1 -> Vehicle Body 3DOF Single Track/4
  Constant3/1 -> Vehicle Body 3DOF Single Track/5
  Constant4/1 -> Vehicle Body 3DOF Single Track/6

== system Model_Slides/Visual Results/Lights and Signs ID ==
  Constant : Constant  Value=TL_ID
  Constant1 : Constant  Value=stopSign_ID
  TL : Outport
  Stop_Sign : Outport  Port=2
  wires:
  Constant/1 -> TL/1
  Constant1/1 -> Stop_Sign/1

== system Model_Slides/Visual Results/Positions and States  ==
  note: Stop Sign positon
  note: Traffic Light Position and State
  <Actors> : Inport
  TL_id : Inport  Port=2
  ss_State : Inport  Port=3
  MATLAB Function1 : MATLAB Function  TreatAsAtomicUnit=on
  MATLAB Function2 : MATLAB Function  TreatAsAtomicUnit=on
  Traffic Light Sensor : Subsystem  mask{TrafficLightSensorModeSelection=Cycle}
      mask prompts: TrafficLightSensorModeSelection "Traffic Light Sensor Mode:"
      mask TypeOptions TrafficLightSensorModeSelection: Steady Green | Steady Red | Cycle
      mask DialogControl DescTextVar Prompt: Simulate a traffic light sensor.
  TL_poses : Outport
  ss_poses : Outport  Port=2
  wires:
  <Actors>/1 -> MATLAB Function2/1(Actors), MATLAB Function1/1(Actors)
  ss_State/1 -> MATLAB Function2/2(ss_State)
  TL_id/1 -> Traffic Light Sensor/1(TL_id)
  Traffic Light Sensor/1(TL_State) -> MATLAB Function1/2(TL_State)  "TL_State"
  MATLAB Function2/1(ss_poses) -> ss_poses/1
  MATLAB Function1/1(TL_poses) -> TL_poses/1

== system Model_Slides/Visual Results/Visualization ==
  note: Visualization
  TL1_poses : Inport
  Actors : Inport  Port=2
  EgoInfo : Inport  Port=3
  ss1_poses : Inport  Port=4
  Visualization : MATLABSystem  System=TL_vis
      mask Type: TL_vis
      mask Display:
      | disp('TL_vis');
      | port_label('input',1,'TL');
      | port_label('input',2,'TargetPoses');
      | port_label('input',3,'EgoInfo');
      | port_label('input',4,'SS');
  wires:
  EgoInfo/1 -> Visualization/3
  Actors/1 -> Visualization/2  "target_vehicle_poses"
  TL1_poses/1 -> Visualization/1
  ss1_poses/1 -> Visualization/4

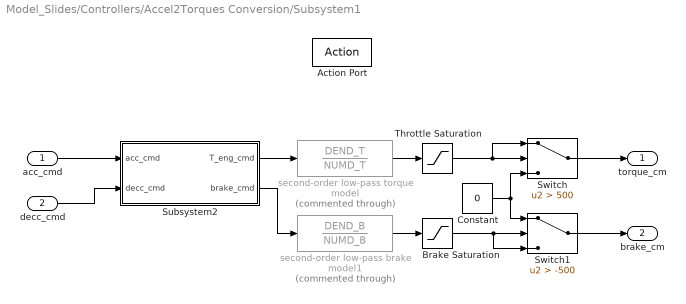
== system Model_Slides/Controllers/Accel2Torques Conversion/Subsystem1 ==
  acc_cmd : Inport
  decc_cmd : Inport  Port=2
  Action Port : ActionPort  ActionPortLabel=case [ 0 ]:
  Brake Saturation : Saturate  UpperLimit=MAX_BRAKE  LowerLimit=MIN_BRAKE
  Constant : Constant  Value=0
  Subsystem2 : Subsystem
  Switch : Switch  Criteria=u2 > Threshold  Threshold=500
  Switch1 : Switch  Criteria=u2 > Threshold  Threshold=-500
  Throttle Saturation : Saturate  UpperLimit=MAX_TORQUE  LowerLimit=MIN_TORQUE
  second-order low-pass brake model1 : DiscreteTransferFcn  Commented=through  Numerator=DEND_B  Denominator=NUMD_B  SampleTime=ts
  second-order low-pass torque model : DiscreteTransferFcn  Commented=through  Numerator=DEND_T  Denominator=NUMD_T  SampleTime=ts
  torque_cm : Outport
  brake_cm : Outport  Port=2
  wires:
  Subsystem2/1(T_eng_cmd) -> second-order low-pass torque model/1
  acc_cmd/1 -> Subsystem2/1(acc_cmd)
  second-order low-pass brake model1/1 -> Brake Saturation/1
  Subsystem2/2(brake_cmd) -> second-order low-pass brake model1/1
  decc_cmd/1 -> Subsystem2/2(decc_cmd)
  second-order low-pass torque model/1 -> Throttle Saturation/1
  Throttle Saturation/1 -> Switch/2, Switch/1
  Switch/1 -> torque_cm/1
  Brake Saturation/1 -> Switch1/2, Switch1/3
  Switch1/1 -> brake_cm/1
  Constant/1 -> Switch/3, Switch1/1

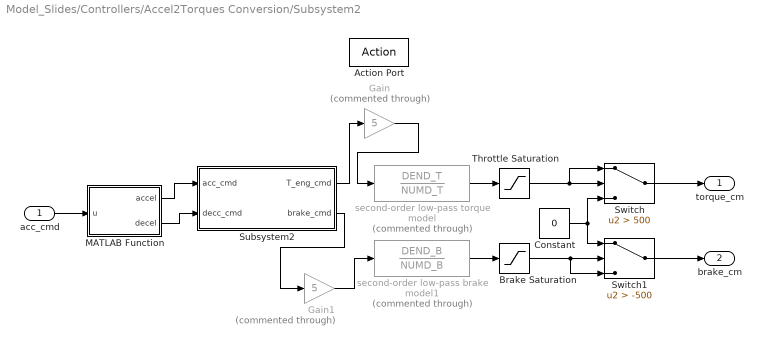
== system Model_Slides/Controllers/Accel2Torques Conversion/Subsystem2 ==
  acc_cmd : Inport
  Action Port : ActionPort  ActionPortLabel=case [ 1 ]:
  Brake Saturation : Saturate  UpperLimit=MAX_BRAKE  LowerLimit=MIN_BRAKE
  Constant : Constant  Value=0
  Gain : Gain  Commented=through  Gain=5
  Gain1 : Gain  Commented=through  Gain=5
  MATLAB Function : MATLAB Function  TreatAsAtomicUnit=on
  Subsystem2 : Subsystem
  Switch : Switch  Criteria=u2 > Threshold  Threshold=500
  Switch1 : Switch  Criteria=u2 > Threshold  Threshold=-500
  Throttle Saturation : Saturate  UpperLimit=MAX_TORQUE  LowerLimit=MIN_TORQUE
  second-order low-pass brake model1 : DiscreteTransferFcn  Commented=through  Numerator=DEND_B  Denominator=NUMD_B  SampleTime=ts
  second-order low-pass torque model : DiscreteTransferFcn  Commented=through  Numerator=DEND_T  Denominator=NUMD_T  SampleTime=ts
  torque_cm : Outport
  brake_cm : Outport  Port=2
  wires:
  second-order low-pass brake model1/1 -> Brake Saturation/1
  second-order low-pass torque model/1 -> Throttle Saturation/1
  Throttle Saturation/1 -> Switch/2, Switch/1
  Switch/1 -> torque_cm/1
  Brake Saturation/1 -> Switch1/2, Switch1/3
  Switch1/1 -> brake_cm/1
  Constant/1 -> Switch/3, Switch1/1
  acc_cmd/1 -> MATLAB Function/1(u)
  MATLAB Function/1(accel) -> Subsystem2/1(acc_cmd)
  MATLAB Function/2(decel) -> Subsystem2/2(decc_cmd)
  Subsystem2/1(T_eng_cmd) -> Gain/1
  Gain/1 -> second-order low-pass torque model/1
  Gain1/1 -> second-order low-pass brake model1/1
  Subsystem2/2(brake_cmd) -> Gain1/1

== system Model_Slides/Reference Data/Theta/thetaBlocks ==
  note: theta calculated from Simulink blocks
  y : Inport
  x : Inport  Port=2
  dis : Inport  Port=3
  Atan2 : Trigonometry  Operator=atan2  ApproximationMethod=CORDIC
  Difference : simulink/Discrete/Difference  ICPrevInput=0.0  OutMin=[]  OutMax=[]  OutDataType=fixdt(1, 16)  OutScaling=2^-10  DoSatur=off
  Difference1 : simulink/Discrete/Difference  ICPrevInput=0.0  OutMin=[]  OutMax=[]  OutDataType=fixdt(1, 16)  OutScaling=2^-10  DoSatur=off
  IC : InitialCondition  Value=psi_o
  Radians to Degrees : simulink_extras/Transformations/Radians to Degrees
  Terminator : Terminator
  theta : Outport
  wires:
  IC/1 -> Radians to Degrees/1
  Atan2/1 -> IC/1
  dis/1 -> Terminator/1
  x/1 -> Difference1/1
  y/1 -> Difference/1
  Radians to Degrees/1 -> theta/1
  Difference/1 -> Atan2/1
  Difference1/1 -> Atan2/2

== system Model_Slides/Reference Data/Theta/thetaLt ==
  note: Check out the script "setUpModel" to understand how we have calculated theta
  note: theta based on lookup table
  y : Inport
  x : Inport  Port=2
  dis : Inport  Port=3
  Terminator : Terminator
  Terminator1 : Terminator
  Theta Ref : Lookup_n-D  NumberOfTableDimensions=1  BreakpointsForDimension1=gradbp  Table=thetaRefs  InternalRulePriority=Speed  RndMeth=Simplest  InputSameDT=on
  theta : Outport
  wires:
  Theta Ref/1 -> theta/1
  dis/1 -> Theta Ref/1
  x/1 -> Terminator1/1
  y/1 -> Terminator/1

== system Model_Slides/Subsystem1/Objects Detection/Tracking ==
  Detections : Inport
  Camera : drivingscenarioandsensors/Vision Detection Generator  SensorIndex=1  DetectorOutput=Objects only  UpdateInterval=0.01  LaneUpdateInterval=0.1  SensorLocation=[1.9 0]  Height=1.1  Yaw=0  Pitch=1  Roll=0  BusNameSource=Auto  BusName=BusObjectDetections  BusName2Source=Auto  BusName2=BusLaneDetections  MaxNumDetectionsSource=Property  MaxNumDetections=10  MaxNumLanesSource=Property  MaxNumLanes=30  DetectionCoordinates=Ego Cartesian  SimulateUsing=Interpreted execution  MaxRange=150  BoundingBoxAccuracy=5  ProcessNoiseIntensity=5  MaxSpeed=100  MaxAllowedOcclusion=0.5  MinObjectImageSize=[1 1]  DetectionProbability=0.9  FalsePositivesPerImage=0.1  MinLaneImageSize=[20 3]  LaneBoundaryAccuracy=3  HasNoise=on  InitialSeedSource=Repeatable  InitialSeed=0  UsedSeed=0  ActorProfilesSource=From Scenario Reader block  ActorProfilesParameters=driving.internal.ActorProfilesParameters  ActorProfilesExpression=[struct('ActorID',1,'ClassID',1,'Length',4.7,'Width',1.8,'Height',1.4,'OriginOffset',[-1.35 0 0],'MeshVertices',[3.7 0.9 0.857439446366782;3.7 -0.9 0.857439446366782;3.7 -0.9 0.314878892733564;3.7 0.9 0.314878892733564;3.7 0.9 0.857439446366782;2.525 0.9 0.993079584775086;2.525 -0.9 0.993079584775086;3.7 -0.9 0.857439446366782;1.82 0.72 1.4;0.41 0.72 1.4;0.41 -0.72 1.4;1.82 -0.72 1.4;-0.295 0.9 0.993079584775086;-1 0.9 0.857439446366782;-1 -0.9 0.857439446366782;-0.295 -0.9 0.993079584775086;3.7 0.9 0.857439446366782;3.7 0.9 0.314878892733564;2.525 0.9 0.314878892733564;2.525 0.9 0.993079584775086;2.525 0.9 0.993079584775086;2.525 0.9 0.314878892733564;-0.295 0.9 0.314878892733564;-0.295 0.9 0.993079584775086;-0.295 0.9 0.993079584775086;-0.295 0.9 0.314878892733564;-1 0.9 0.355570934256055;-1 0.9 0.857439446366782;2.525 0.9 0.993079584775086;-0.295 0.9 0.993079584775086;0.41 0.72 1.4;1.82 0.72 1.4;3.7 -0.9 0.857439446366782;3.7 -0.9 0.314878892733564;2.525 -0.9 0.314878892733564;2.525 -0.9 0.993079584775086;2.525 -0.9 0.993079584775086;2.525 -0.9 0.314878892733564;-0.295 -0.9 0.314878892733564;-0.295 -0.9 0.993079584775086;-0.295 -0.9 0.993079584775086;-0.295 -0.9 0.314878892733564;-1 -0.9 0.355570934256055;-1 -0.9 0.857439446366782;2.525 -0.9 0.993079584775086;-0.295 -0.9 0.993079584775086;0.41 -0.72 1.4;1.82 -0.72 1.4;-0.295 0.9 0.993079584775086;-0.295 -0.9 0.993079584775086;0.41 -0.72 1.4;0.41 0.72 1.4;2.525 -0.9 0.993079584775086;1.82 -0.72 1.4;1.82 0.72 1.4;2.525 0.9 0.993079584775086;-1 0.9 0.857439446366782;-1 0.9 0.355570934256055;-1 -0.9 0.355570934256055;-1 -0.9 0.857439446366782;3.7 0.9 0.314878892733564;3.7 -0.9 0.314878892733564;-0.295 -0.9 0.314878892733564;-0.295 0.9 0.314878892733564;-0.295 0.9 0.314878892733564;-1 0.9 0.355570934256055;-1 -0.9 0.355570934256055;-0.295 -0.9 0.314878892733564;0 -0.63 0;0 -0.87 0;0.191030206995054 -0.63 0.0601365173421445;0.191030206995054 -0.87 0.0601365173421445;0.309093367795925 -0.63 0.217575963708927;0.309093367795925 -0.87 0.217575963708927;0.309093367795925 -0.63 0.412181821758201;0.309093367795925 -0.87 0.412181821758201;0.191030206995054 -0.63 0.569621268124983;0.191030206995054 -0.87 0.569621268124983;0 -0.63 0.629757785467128;0 -0.87 0.629757785467128;-0.191030206995054 -0.63 0.569621268124983;-0.191030206995054 -0.87 0.569621268124983;-0.309093367795925 -0.63 0.412181821758201;-0.309093367795925 -0.87 0.412181821758201;-0.309093367795925 -0.63 0.217575963708927;-0.309093367795925 -0.87 0.217575963708927;-0.191030206995054 -0.63 0.0601365173421445;-0.191030206995054 -0.87 0.0601365173421445;0 -0.63 0;0 -0.87 0;0 -0.63 0;0.191030206995054 -0.63 0.0601365173421445;0.309093367795925 -0.63 0.217575963708927;0.309093367795925 -0.63 0.412181821758201;0.191030206995054 -0.63 0.569621268124983;0 -0.63 0.629757785467128;-0.191030206995054 -0.63 0.569621268124983;-0.309093367795925 -0.63 0.412181821758201;-0.309093367795925 -0.63 0.217575963708927;-0.191030206995054 -0.63 0.0601365173421445;0 -0.87 0;0.191030206995054 -0.87 0.0601365173421445;0.309093367795925 -0.87 0.217575963708927;0.309093367795925 -0.87 0.412181821758201;0.191030206995054 -0.87 0.569621268124983;0 -0.87 0.629757785467128;-0.191030206995054 -0.87 0.569621268124983;-0.309093367795925 -0.87 0.412181821758201;-0.309093367795925 -0.87 0.217575963708927;-0.191030206995054 -0.87 0.0601365173421445;0 0.87 0;0 0.63 0;0.191030206995054 0.87 0.0601365173421445;0.191030206995054 0.63 0.0601365173421445;0.309093367795925 0.87 0.217575963708927;0.309093367795925 0.63 0.217575963708927;0.309093367795925 0.87 0.412181821758201;0.309093367795925 0.63 0.412181821758201;0.191030206995054 0.87 0.569621268124983;0.191030206995054 0.63 0.569621268124983;0 0.87 0.629757785467128;0 0.63 0.629757785467128;-0.191030206995054 0.87 0.569621268124983;-0.191030206995054 0.63 0.569621268124983;-0.309093367795925 0.87 0.412181821758201;-0.309093367795925 0.63 0.412181821758201;-0.309093367795925 0.87 0.217575963708927;-0.309093367795925 0.63 0.217575963708927;-0.191030206995054 0.87 0.0601365173421445;-0.191030206995054 0.63 0.0601365173421445;0 ...(+3718 chars)],'MeshFaces',[1 2 3;3 4 1;5 6 7;7 8 5;9 10 11;11 12 9;13 14 15;15 16 13;17 18 19;19 20 17;21 22 23;23 24 21;25 26 27;27 28 25;29 30 31;31 32 29;33 34 35;35 36 33;37 38 39;39 40 37;41 42 43;43 44 41;45 46 47;47 48 45;49 50 51;51 52 49;53 54 55;55 56 53;57 58 59;59 60 57;61 62 63;63 64 61;65 66 67;67 68 65;69 71 72;72 70 69;71 73 74;74 72 71;73 75 76;76 74 73;75 77 78;78 76 75;77 79 80;80 78 77;79 81 82;82 80 79;81 83 84;84 82 81;83 85 86;86 84 83;85 87 88;88 86 85;87 89 90;90 88 87;91 92 93;91 93 94;91 94 95;91 95 96;91 96 97;91 97 98;91 98 99;91 99 100;101 102 103;101 103 104;101 104 105;101 105 106;101 106 107;101 107 108;101 108 109;101 109 110;111 113 114;114 112 111;113 115 116;116 114 113;115 117 118;118 116 115;117 119 120;120 118 117;119 121 122;122 120 119;121 123 124;124 122 121;123 125 126;126 124 123;125 127 128;128 126 125;127 129 130;130 128 127;129 131 132;132 130 129;133 134 135;133 135 136;133 136 137;133 137 138;133 138 139;133 139 140;133 140 141;133 141 142;143 144 145;143 145 146;143 146 147;143 147 148;143 148 149;143 149 150;143 150 151;143 151 152;153 155 156;156 154 153;155 157 158;158 156 155;157 159 160;160 158 157;159 161 162;162 160 159;161 163 164;164 162 161;163 165 166;166 164 163;165 167 168;168 166 165;167 169 170;170 168 167;169 171 172;172 170 169;171 173 174;174 172 171;175 176 177;175 177 178;175 178 179;175 179 180;175 180 181;175 181 182;175 182 183;175 183 184;185 186 187;185 187 188;185 188 189;185 189 190;185 190 191;185 191 192;185 192 193;185 193 194;195 197 198;198 196 195;197 199 200;200 198 197;199 201 202;202 200 199;201 203 204;204 202 201;203 205 206;206 204 203;205 207 208;208 206 205;207 209 210;210 208 207;209 211 212;212 210 209;211 213 214;214 212 211;213 215 216;216 214 213;217 218 219;217 219 220;217 220 221;217 221 222;217 222 223;217 223 224;217 224 225;217 225 226;227 228 229;227 229 230;227 230 231;227 231 232;227 232 233;227 233 234;227 234 235;227 235 236],'RCSPattern',[10 10;10 10],'RCSAzimuthAngles',[-180 180],'RCSElevationAngles',[-90 90]); struct('ActorID',2,'ClassID',7,'Length',0.7,'Width',0.2,'Height',0.1,'OriginOffset',[0 0 0],'MeshVertices',[0.35 -0.1 0.1;0.35 0.1 0.1;-0.35 0.1 0.1;-0.35 -0.1 0.1;0.35 -0.1 0;0.35 0.1 0;-0.35 0.1 0;-0.35 -0.1 0],'MeshFaces',[6 2 1;1 5 6;8 4 3;3 7 8;6 7 3;3 2 6;5 1 4;4 8 5;4 1 2;2 3 4;7 6 5;5 8 7],'RCSPattern',[10 10;10 10],'RCSAzimuthAngles',[-180 180],'RCSElevationAngles',[-90 90])]  Intrinsics=driving.internal.cameraIntrinsics('FocalLength',[400 800],'PrincipalPoint',[320 240],'ImageSize',[480 640],'RadialDistortion',[0 0],'TangentialDistortion',[0 0],'Skew',0)
  Detection Concatenation : trackingutilitieslib/Detection Concatenation  NumInputs=2  BusNameSource=Property  BusName=Detections  SimulateUsing=Interpreted execution
      settings: SourceProductBaseCode=AE,DR,TF,RA,UV,VE
  Multi-Object Tracker : drivinglib/Multi-Object Tracker  TrackerIndex=uint32( 0 )  FilterInitializationFcn=helperInitSimulinkDemoFilter  AssignmentThreshold=50  ConfirmationThreshold=[ 2, 3 ]  DeletionThreshold=[ 5, 5 ]  MaxNumTracks=20  MaxNumSensors=20  OOSMHandling=Neglect  StateParametersSimulink=struct  HasStateParametersInput=off  TimeInputSource=Auto  HasCostMatrixInput=off  HasDetectableTrackIDsInput=off  BusNameSource=Auto  BusName=BusMultiObjectTracker  TentativeTracksOutputPort=off  AllTracksOutputPort=off  SimulateUsing=Interpreted execution
      settings: SourceProductBaseCode=DR
  Radar Detection Generator : drivingscenarioandsensors/Radar Detection Generator  SensorIndex=2  UpdateInterval=0.01  SensorLocation=[ 1.5, 0 ]  Height=0.2  Yaw=0  Pitch=0  Roll=0  BusNameSource=Auto  BusName=BusRadarDetectionGenerator  MaxNumDetectionsSource=Property  MaxNumDetections=50  DetectionCoordinates=Ego Cartesian  SimulateUsing=Interpreted execution  AzimuthResolution=4  ElevationResolution=10  RangeResolution=2.5  RangeRateResolution=0.5  AzimuthBiasFraction=0.1  ElevationBiasFraction=0.1  RangeBiasFraction=0.05  RangeRateBiasFraction=0.05  FieldOfView=[ 60, 5 ]  MaxRange=150  RangeRateLimits=[ -100, 100 ]  DetectionProbability=0.9  FalseAlarmRate=1e-6  ReferenceRange=100  ReferenceRCS=0  HasElevation=off  HasRangeRate=on  HasNoise=on  HasFalseAlarms=on  HasOcclusion=on  InitialSeedSource=Repeatable  InitialSeed=0  UsedSeed=matlabshared.tracking.internal.SimulinkUtilities.seedManager(gcb)  ActorProfilesSource=Parameters  ActorProfilesParameters=driving.internal.ActorProfilesRadarParameters  ActorProfilesExpression=struct( 'ClassID', 0, 'Length', 4.7, 'Width', 1.8, 'Height', 1.4, 'OriginOffset', [ -1.35, 0, 0 ], 'RCSPattern', [ 10, 10; 10, 10 ], 'RCSAzimuthAngles', [ -180, 180 ], 'RCSElevationAngles', [ -90, 90 ] )
      settings: SourceProductBaseCode=DR
  Subsystem1 : Subsystem  Commented=on
  Confirmed_Tracks : Outport
  wires:
  Camera/1 -> Detection Concatenation/1  "Camera Detections"
  Radar Detection Generator/1 -> Detection Concatenation/2  "Lidar Detections"
  Detections/1 -> Radar Detection Generator/1, Camera/1
  Detection Concatenation/1 -> Multi-Object Tracker/1
  Multi-Object Tracker/1 -> Confirmed_Tracks/1

== system Model_Slides/Vehicle Dynamics1/Subsystem/Signal Builder ==
  Demux : Demux  Tag=STV Demux  Outputs=3
      settings: DisplayOption=none
  FromWs : FromWorkspace  Tag=STV FromWs  VariableName=tuvar
      SigBuilderData=|
      | common.afterFinalStr = 'Extrapolate'
      | common.sampleTime = 0
      | dataSet.timeRange = [0 3.5]
      | dataSet.name = 'DriveAndTurn'
      | sbobj.Groups.Name = 'DriveAndTurn'
      | sbobj.Groups.Signals(1).Name = 'Normalized Torque'
      | sbobj.Groups.Signals(1).XData = [0 1 1 2 2 3.5]
      | sbobj.Groups.Signals(1).YData = [1 1 0 0 1 1]
      | sbobj.Groups.Signals(2).Name = 'Normalized Brake'
      | sbobj.Groups.Signals(2).XData = [0 1 1 2 2 3.5]
      | sbobj.Groups.Signals(2).YData = [0 0 1 1 0 0]
      | sbobj.Groups.Signals(3).Name = 'Normalized Steer'
      | sbobj.Groups.Signals(3).XData = [0 0.5 0.6 1.02 1.02 2 2.5 3 3.5]
      | sbobj.Groups.Signals(3).YData = [-0.02 -0.02 -0.02 -0.3 -1.02 -0.92 -0.34 0.14 0.22]
      | sbobj.Groups.TimeRange = [0 3.5]
  Normalized Torque : Outport  Tag=STV Outport
  Normalized Brake : Outport  Tag=STV Outport  Port=2
  Normalized Steer : Outport  Tag=STV Outport  Port=3
  wires:
  FromWs/1 -> Demux/1
  Demux/1 -> Normalized Torque/1
  Demux/2 -> Normalized Brake/1
  Demux/3 -> Normalized Steer/1
